simulink model "Dron_no_lineal"  (R2022a)
settings: Solver=VariableStepAuto  StartTime=0.0  StopTime=10  FixedStep=Ts  RelTol=1e-3
PreLoadFcn:
  | parametros
undefined symbols (not defined in the file): g, Ix, Iy, Iz, Kt, l, m
libraries: simulink x3
settings Model: Creator=juani  LastModifiedBy=juani
settings SolverCC: MaxConsecutiveMinStep=100  ZeroCrossAlgorithm=Adaptive
settings DebuggingCC: MaskedZcDiagnostic=none  IgnoredZcDiagnostic=none

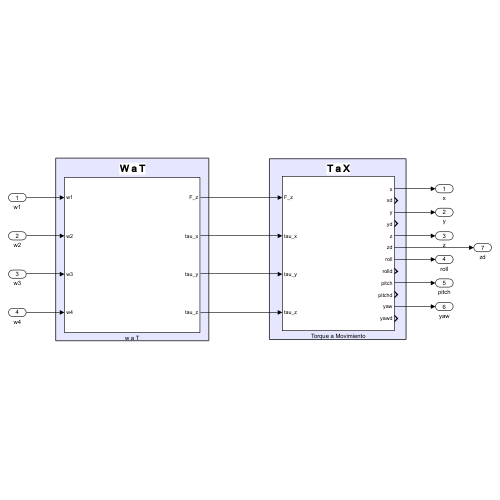
[thumbnail: Simulink's stored preview of the top-level diagram]
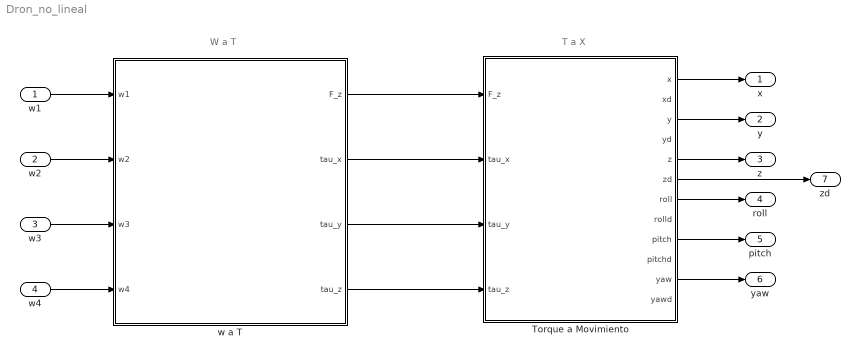
== system Dron_no_lineal ==
  note: W a T
  note: T a X
  w1 : Inport
  w2 : Inport  Port=2
  w3 : Inport  Port=3
  w4 : Inport  Port=4
  Torque a Movimiento : Subsystem
  w a T : Subsystem
  x : Outport
  y : Outport  Port=2
  z : Outport  Port=3
  roll : Outport  Port=4
  pitch : Outport  Port=5
  yaw : Outport  Port=6
  zd : Outport  Port=7
  wires:
  Torque a Movimiento/1(x) -> x/1
  Torque a Movimiento/3(y) -> y/1
  Torque a Movimiento/5(z) -> z/1
  Torque a Movimiento/7(roll) -> roll/1
  Torque a Movimiento/9(pitch) -> pitch/1
  Torque a Movimiento/11(yaw) -> yaw/1
  Torque a Movimiento/6(zd) -> zd/1
  w4/1 -> w a T/4(w4)
  w2/1 -> w a T/2(w2)
  w1/1 -> w a T/1(w1)
  w3/1 -> w a T/3(w3)
  w a T/1(F_z) -> Torque a Movimiento/1(F_z)
  w a T/2(tau_x) -> Torque a Movimiento/2(tau_x)
  w a T/3(tau_y) -> Torque a Movimiento/3(tau_y)
  w a T/4(tau_z) -> Torque a Movimiento/4(tau_z)

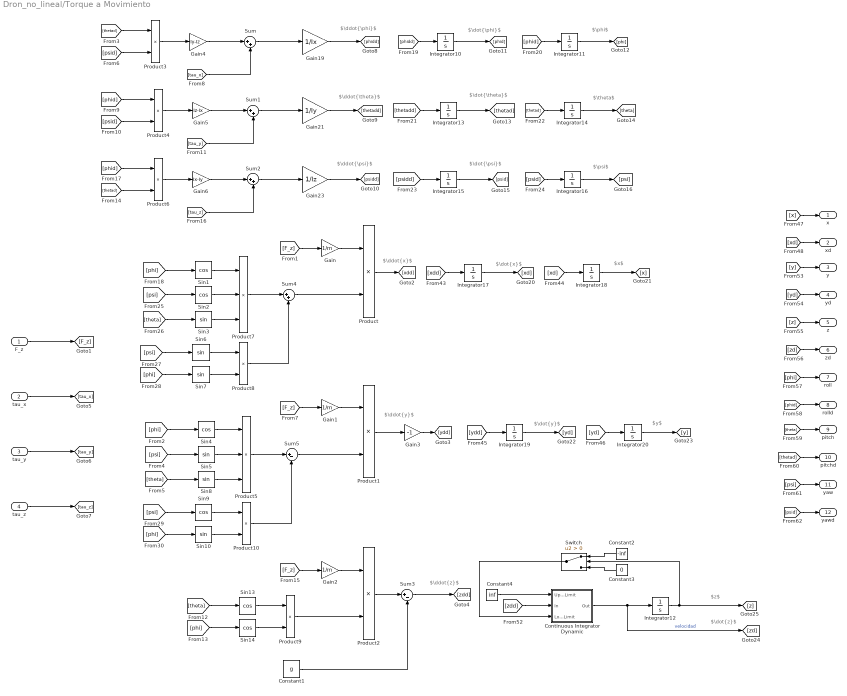
== system Dron_no_lineal/Torque a Movimiento ==
  note: $\ddot{x}$
  note: $\theta$
  note: $\dot{\psi}$
  note: $\dot{y}$
  note: $\ddot{z}$
  note: $\dot{\phi}$
  note: $\phi$
  note: $\dot{\theta}$
  note: $\psi$
  note: $z$
  note: $x$
  note: $\ddot{\phi}$
  note: $\dot{x}$
  note: $y$
  note: $\dot{z}$
  note: $\ddot{y}$
  note: $\ddot{\psi}$
  note: $\ddot{\theta}$
  F_z : Inport
  tau_x : Inport  Port=2
  tau_y : Inport  Port=3
  tau_z : Inport  Port=4
  Constant1 : Constant  Value=g
  Constant2 : Constant  Value=-inf
  Constant3 : Constant  Value=0
  Constant4 : Constant  Value=inf
  Continuous Integrator Dynamic : Subsystem
  Gain : Gain  Gain=1/m
  Gain1 : Gain  Gain=1/m
  Gain19 : Gain  Gain=1/Ix
  Gain2 : Gain  Gain=1/m
  Gain21 : Gain  Gain=1/Iy
  Gain23 : Gain  Gain=1/Iz
  Gain3 : Gain  Gain=-1
  Gain4 : Gain  Gain=Iy-Iz
  Gain5 : Gain  Gain=Iz-Ix
  Gain6 : Gain  Gain=Ix-Iy
  Integrator{10..11,13..20} (10 alike) : Integrator
  Integrator12 : Integrator  LimitOutput=on  LowerSaturationLimit=0
  Product{,1..4,6,8..10} (9 alike) : Product
  Product5 : Product  Inputs=3
  Product7 : Product  Inputs=3
  Sin{1..2,4,9,13..14} (6 alike) : Trigonometry  Operator=cos
  Sin{3,5..8,10} (6 alike) : Trigonometry
  Sum{,1..2,4} (4 alike) : Sum  Inputs=|++
  Sum3 : Sum  Inputs=|+-
  Sum5 : Sum  Inputs=|+-
  Switch : Switch  Criteria=u2 > Threshold  SaturateOnIntegerOverflow=off  InputSameDT=off
  x : Outport
  xd : Outport  Port=2
  y : Outport  Port=3
  yd : Outport  Port=4
  z : Outport  Port=5
  zd : Outport  Port=6
  roll : Outport  Port=7
  rolld : Outport  Port=8
  pitch : Outport  Port=9
  pitchd : Outport  Port=10
  yaw : Outport  Port=11
  yawd : Outport  Port=12
  wires:
  [phi] -> Sin4/1
  [zdd] -> Continuous Integrator Dynamic/2(In)
  [phidd] -> Integrator10/1
  Sin5/1 -> Product5/2
  Sin3/1 -> Product7/3
  [xdd] -> Integrator17/1
  [phi] -> Sin10/1
  [theta] -> pitch/1
  tau_z/1 -> [tau_z]
  [phid] -> Integrator11/1
  Product1/1 -> Gain3/1
  Sin4/1 -> Product5/1
  Sin7/1 -> Product8/2
  [psi] -> Sin2/1
  Product7/1 -> Sum4/1
  [theta] -> Sin8/1
  Sin10/1 -> Product10/2
  [tau_z] -> Sum2/2
  [zd] -> zd/1
  Gain3/1 -> [ydd]
  [psi] -> Sin9/1
  [thetad] -> Integrator14/1
  [thetadd] -> Integrator13/1
  Product8/1 -> Sum4/2
  Product9/1 -> Product2/2
  Sum5/1 -> Product1/2
  Gain2/1 -> Product2/1
  Sum2/1 -> Gain23/1
  [psi] -> Sin6/1
  Sin8/1 -> Product5/3
  Sin9/1 -> Product10/1
  Product10/1 -> Sum5/2
  Sin6/1 -> Product8/1
  [psi] -> Sin5/1
  [theta] -> Sin13/1
  Constant4/1 -> Continuous Integrator Dynamic/1(Upper Limit)
  Integrator11/1 -> [phi]
  [phid] -> Product4/1
  Sin1/1 -> Product7/1
  Sum4/1 -> Product/2
  [phi] -> Sin7/1
  [thetad] -> Product6/2
  Sin13/1 -> Product9/1
  [theta] -> Sin3/1
  [y] -> y/1
  Sin2/1 -> Product7/2
  Product2/1 -> Sum3/1
  Product6/1 -> Gain6/1
  Gain4/1 -> Sum/1
  Gain6/1 -> Sum2/1
  Sum1/1 -> Gain21/1
  [psid] -> Product4/2
  Product4/1 -> Gain5/1
  [tau_x] -> Sum/2
  Gain/1 -> Product/1
  Product3/1 -> Gain4/1
  [thetad] -> Product3/1
  Product/1 -> [xdd]
  [ydd] -> Integrator19/1
  Constant1/1 -> Sum3/2
  Gain5/1 -> Sum1/1
  [tau_y] -> Sum1/2
  Sin14/1 -> Product9/2
  Integrator12/1 -> [z], Switch/2
  [F_z] -> Gain1/1
  Gain23/1 -> [psidd]
  [psid] -> yawd/1
  [phi] -> roll/1
  tau_x/1 -> [tau_x]
  [psid] -> Integrator16/1
  Integrator14/1 -> [theta]
  [xd] -> xd/1
  [x] -> x/1
  [F_z] -> Gain/1
  F_z/1 -> [F_z]
  [psidd] -> Integrator15/1
  [psi] -> yaw/1
  [psid] -> Product3/2
  [phi] -> Sin1/1
  [z] -> z/1
  Integrator13/1 -> [thetad]
  tau_y/1 -> [tau_y]
  Gain1/1 -> Product1/1
  [phid] -> rolld/1
  Integrator16/1 -> [psi]
  Integrator10/1 -> [phid]
  [yd] -> Integrator20/1
  Sum3/1 -> [zdd]
  Constant2/1 -> Switch/1
  Continuous Integrator Dynamic/1(Out) -> [zd], Integrator12/1  "velocidad"
  [phi] -> Sin14/1
  Gain19/1 -> [phidd]
  Integrator18/1 -> [x]
  [xd] -> Integrator18/1
  Sum/1 -> Gain19/1
  Gain21/1 -> [thetadd]
  [yd] -> yd/1
  Product5/1 -> Sum5/1
  Switch/1 -> Continuous Integrator Dynamic/3(Lower Limit)
  Integrator20/1 -> [y]
  [F_z] -> Gain2/1
  [phid] -> Product6/1
  Constant3/1 -> Switch/3
  Integrator15/1 -> [psid]
  [thetad] -> pitchd/1
  Integrator17/1 -> [xd]
  Integrator19/1 -> [yd]

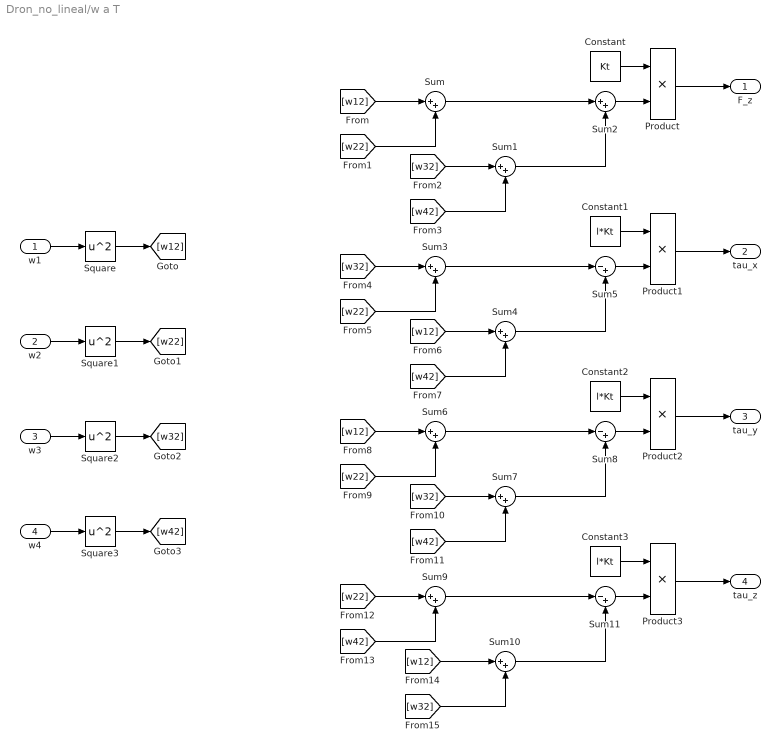
== system Dron_no_lineal/w a T ==
  w1 : Inport
  w2 : Inport  Port=2
  w3 : Inport  Port=3
  w4 : Inport  Port=4
  Constant : Constant  Value=Kt
  Constant1 : Constant  Value=l*Kt
  Constant2 : Constant  Value=l*Kt
  Constant3 : Constant  Value=l*Kt
  Product{,1..3} (4 alike) : Product
  Square{,1..3} (4 alike) : Math  Operator=square
  Sum{,1..4,6..7,9..10} (9 alike) : Sum  Inputs=|++
  Sum11 : Sum  Inputs=|-+
  Sum5 : Sum  Inputs=|-+
  Sum8 : Sum  Inputs=|-+
  F_z : Outport
  tau_x : Outport  Port=2
  tau_y : Outport  Port=3
  tau_z : Outport  Port=4
  wires:
  Product2/1 -> tau_y/1
  [w12] -> Sum6/1
  [w22] -> Sum9/1
  Constant/1 -> Product/1
  Sum9/1 -> Sum11/1
  [w22] -> Sum6/2
  Product/1 -> F_z/1
  Sum6/1 -> Sum8/1
  [w32] -> Sum10/2
  [w32] -> Sum7/1
  Sum7/1 -> Sum8/2
  Square2/1 -> [w32]
  Square1/1 -> [w22]
  [w42] -> Sum7/2
  Square/1 -> [w12]
  Product1/1 -> tau_x/1
  Sum2/1 -> Product/2
  [w32] -> Sum3/1
  Sum3/1 -> Sum5/1
  [w32] -> Sum1/1
  Sum1/1 -> Sum2/2
  Product3/1 -> tau_z/1
  Sum10/1 -> Sum11/2
  [w42] -> Sum9/2
  Square3/1 -> [w42]
  Sum5/1 -> Product1/2
  [w42] -> Sum4/2
  Constant1/1 -> Product1/1
  [w22] -> Sum/2
  Sum/1 -> Sum2/1
  [w12] -> Sum/1
  w1/1 -> Square/1
  [w12] -> Sum4/1
  w2/1 -> Square1/1
  w3/1 -> Square2/1
  [w12] -> Sum10/1
  [w42] -> Sum1/2
  Sum11/1 -> Product3/2
  Sum4/1 -> Sum5/2
  Sum8/1 -> Product2/2
  Constant3/1 -> Product3/1
  Constant2/1 -> Product2/1
  [w22] -> Sum3/2
  w4/1 -> Square3/1

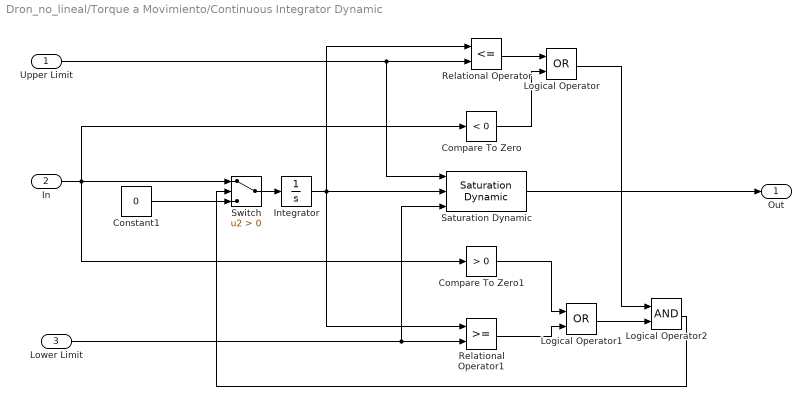
== system Dron_no_lineal/Torque a Movimiento/Continuous Integrator Dynamic ==
  Upper Limit : Inport
  In : Inport  Port=2
  Lower Limit : Inport  Port=3
  Compare To Zero : simulink/Logic and Bit Operations/Compare To Zero  relop=<  OutDataTypeStr=uint8  ZeroCross=off
  Compare To Zero1 : simulink/Logic and Bit Operations/Compare To Zero  relop=>  OutDataTypeStr=uint8  ZeroCross=off
  Constant1 : Constant  Value=0
  Integrator : Integrator
  Logical Operator : Logic  Operator=OR  AllPortsSameDT=off  OutDataTypeStr=boolean
  Logical Operator1 : Logic  Operator=OR  AllPortsSameDT=off  OutDataTypeStr=boolean
  Logical Operator2 : Logic  AllPortsSameDT=off  OutDataTypeStr=boolean
  Relational Operator : RelationalOperator  Operator=<=  OutDataTypeStr=boolean  InputSameDT=off
  Relational Operator1 : RelationalOperator  OutDataTypeStr=boolean  InputSameDT=off
  Saturation Dynamic : simulink/Discontinuities/Saturation Dynamic  OutMin=[]  OutMax=[]  OutDataTypeStr=Inherit: Same as second input  OutDataType=fixdt(1, 16)  OutScaling=2^-10  DoSatur=off
  Switch : Switch  Criteria=u2 > Threshold  SaturateOnIntegerOverflow=off  InputSameDT=off
  Out : Outport  VectorParamsAs1DForOutWhenUnconnected=off
  wires:
  In/1 -> Compare To Zero/1, Compare To Zero1/1, Switch/1
  Constant1/1 -> Switch/3
  Switch/1 -> Integrator/1
  Relational Operator/1 -> Logical Operator/1
  Compare To Zero/1 -> Logical Operator/2
  Upper Limit/1 -> Relational Operator/2, Saturation Dynamic/1
  Lower Limit/1 -> Relational Operator1/2, Saturation Dynamic/3
  Compare To Zero1/1 -> Logical Operator1/1
  Relational Operator1/1 -> Logical Operator1/2
  Logical Operator1/1 -> Logical Operator2/2
  Logical Operator/1 -> Logical Operator2/1
  Logical Operator2/1 -> Switch/2
  Saturation Dynamic/1 -> Out/1
  Integrator/1 -> Relational Operator/1, Relational Operator1/1, Saturation Dynamic/2
